simulink subsystem "quatquad_dynamics_sim"  (R2021b)
settings: Solver=VariableStepAuto  StartTime=0.0  StopTime=10.0  RelTol=1e-3
values from neighbouring files (symbols this model uses):
  x_0 = x_r(:,1)    [quatquad_main.m]
libraries: sharedutil x1
settings Model: Creator=vifre  LastModifiedBy=vifre

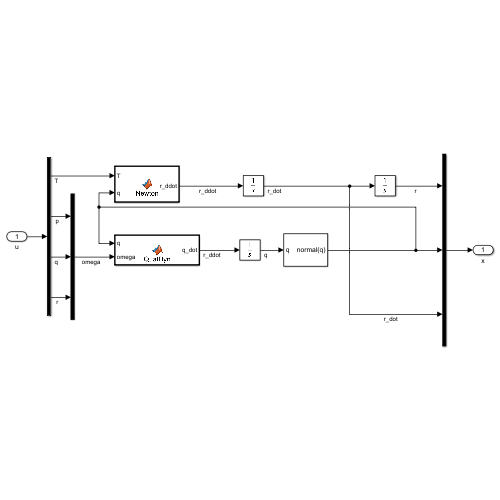
[thumbnail: Simulink's stored preview of the top-level diagram]
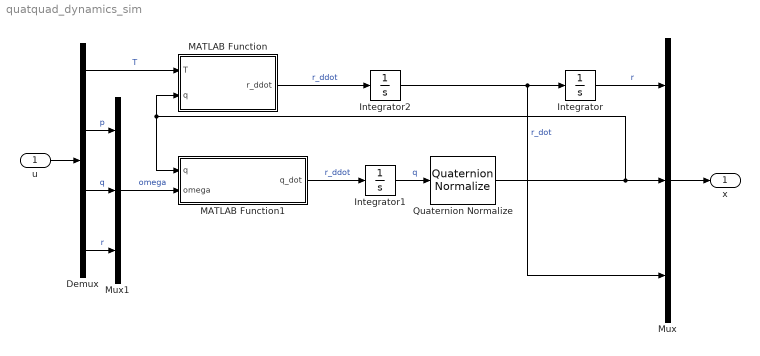
== system quatquad_dynamics_sim ==
  u : Inport
  Demux : Demux
  Integrator : Integrator  InitialCondition=x_0(1:3)
  Integrator1 : Integrator  InitialCondition=x_0(4:7)
  Integrator2 : Integrator  InitialCondition=x_0(8:10)
  MATLAB Function : MATLAB Function  TreatAsAtomicUnit=on
  MATLAB Function1 : MATLAB Function  TreatAsAtomicUnit=on
  Mux : Mux  Inputs=3
  Mux1 : Mux  Inputs=3
  Quaternion Normalize : sharedutil/Quaternion Normalize  aMode=aMode
      settings: SourceProductBaseCode=AE,PW,DR,MT,UV,VE
  x : Outport
  wires:
  Demux/2 -> Mux1/1  "p"
  Mux/1 -> x/1
  Mux1/1 -> MATLAB Function1/2(omega)  "omega"
  Demux/3 -> Mux1/2  "q"
  Demux/1 -> MATLAB Function/1(T)  "T"
  MATLAB Function/1(r_ddot) -> Integrator2/1  "r_ddot"
  Integrator2/1 -> Mux/3, Integrator/1  "r_dot"
  Integrator1/1 -> Quaternion Normalize/1  "q"
  u/1 -> Demux/1
  Quaternion Normalize/1 -> MATLAB Function/2(q), MATLAB Function1/1(q), Mux/2
  Demux/4 -> Mux1/3  "r"
  MATLAB Function1/1(q_dot) -> Integrator1/1  "r_ddot"
  Integrator/1 -> Mux/1  "r"

== matlab function quatquad_dynamics_sim/MATLAB Function ==
  data: T input; r_ddot output; q input
function r_ddot = Newton(T,q)
x_ddot = 2*T*(q(1)*q(3) + q(2)*q(4));
y_ddot = -2*T*(q(1)*q(2) - q(3)*q(4));
z_ddot = T*(q(1)^2 - q(2)^2 - q(3)^2 + q(4)^2) - 9.81;
r_ddot = [x_ddot;y_ddot;z_ddot];
end

== matlab function quatquad_dynamics_sim/MATLAB Function1 ==
  data: q input; omega input; q_dot output
function q_dot = QuatDyn(q,omega)
q_dot = zeros(4,1);
q_dot(1) =  - (omega(1)*q(2))/2 - (omega(2)*q(3))/2 - (omega(3)*q(4))/2;
q_dot(2) =    (omega(1)*q(1))/2 - (omega(2)*q(4))/2 + (omega(3)*q(3))/2;
q_dot(3) =    (omega(1)*q(4))/2 + (omega(2)*q(1))/2 - (omega(3)*q(2))/2;
q_dot(4) =  - (omega(1)*q(3))/2 + (omega(2)*q(2))/2 + (omega(3)*q(1))/2;
end
